simulink model "Copy_of_WorkshopB_1"  (R2014b)
settings: Solver=ode45  SolverMode=SingleTasking  StartTime=0.0  StopTime=5  RelTol=1e-3
values from neighbouring files (symbols this model uses):
  dm = dm*eps_dm    (= 1.3528e-05)    [param.m]
  Dpos = double(D)    [param.m]
  Fc = 0.0013    [param.m]
  Ipos = double(I)    [param.m]
  Jeq = eps_Jeq*Jeq    (= 2.20476e-05)    [param.m]
  Kemf = 1/(137*2*pi/60)    (= 0.0697028947848)    [param.m]
  Km = 69.7E-3    (= 0.0697)    [param.m]
  Max_Accel = Km*MaxCurrent/Jeq    (= 460.291369582)    [param.m]
  Max_Speed = MaxVoltage/Kemf    (= 275.454843867)    [param.m]
  n = 1    [param.m]
  Npos = double(N)    [param.m]
  Ppos = double(P)    [param.m]
  R = s*s + s*N    [PID_calc.m]    (also in param.m = 112)
  Ts = 5e-3    (= 0.005)    [param.m]
undefined symbols (not defined in the file or in its folder): sigbuilder_block
settings Model: Creator=sofianh  LastModifiedBy=es2lab2
settings OptimizationCC: BlockReduction=off  BooleanDataType=off  UseDivisionForNetSlopeComputation=off  SimCompilerOptimization=off
settings DebuggingCC: SaveWithParameterizedLinksMsg=none  UnderspecifiedInitializationDetection=Classic  MergeDetectMultiDrivingBlocksExec=none  SignalResolutionControl=TryResolveAllWithWarning  SolverPrmCheckMsg=none  FrameProcessingCompatibilityMsg=error  AllowSymbolicDim=off
settings HardwareCC: TargetUnknown=on
settings RTWCC: RTWCompilerOptimization=off
settings ConfigComp: CovMetricSettings=dw  CovHtmlReporting=on  CovSaveCumulativeToWorkspaceVar=on  CovSaveSingleToWorkspaceVar=on  CovModelRefEnable=Off  CovExternalEMLEnable=off  CovSFcnEnable=off

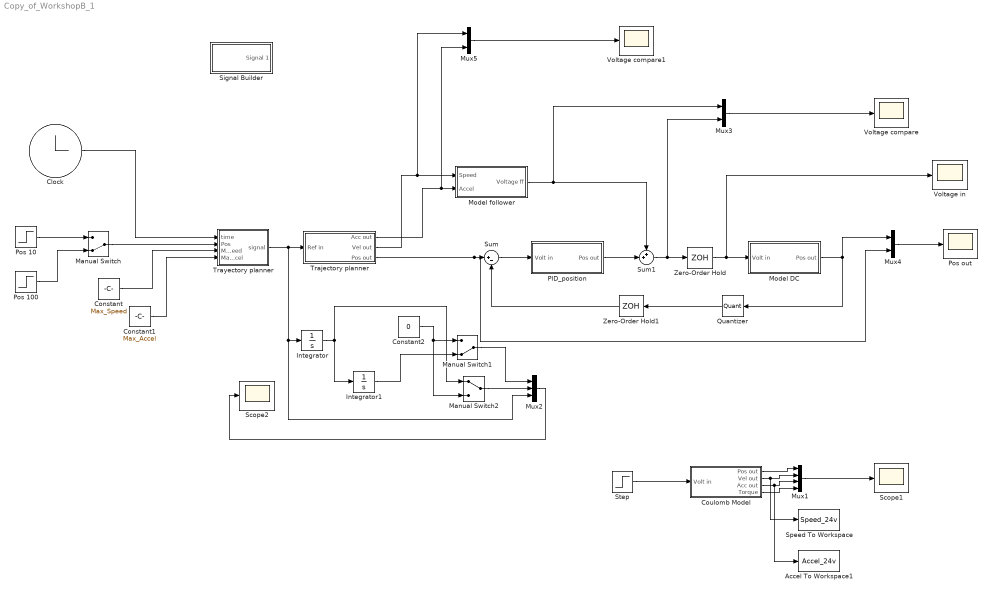
== system Copy_of_WorkshopB_1 ==
  Accel To Workspace1 : ToWorkspace  VariableName=Accel_24v  SaveFormat=Timeseries  SampleTime=-1
  Clock : Clock
  Constant : Constant  Value=Max_Speed
  Constant1 : Constant  Value=Max_Accel
  Constant2 : Constant  Value=0
  Coulomb Model : Subsystem
  Integrator : Integrator
  Integrator1 : Integrator
  Manual Switch : ManualSwitch  CurrentSetting=0
  Manual Switch1 : ManualSwitch  CurrentSetting=0
  Manual Switch2 : ManualSwitch
  "Model DC " : Subsystem
  Model follower : Subsystem
  Mux1 : Mux
  Mux2 : Mux  Inputs=3
  Mux3 : Mux  Inputs=2
  Mux4 : Mux  Inputs=2
  Mux5 : Mux  Inputs=2
  PID_position : Subsystem
  Pos 10 : Step  Time=0  After=10  SampleTime=0
  Pos 100 : Step  Time=0  After=100  SampleTime=0
  Pos out : Scope
      settings: TimeRange=4  SaveName=ScopeData3
  Quantizer : Quantizer  QuantizationInterval=Pulses  SampleTime=Ts
  Scope1 : Scope
  Scope2 : Scope
      settings: TimeRange=1  YMin=0  YMax=450
  Signal Builder : Subsystem  Tag=STV Subsys  LoadFcn=sigbuilder_block('load');  StartFcn=sigbuilder_block('start');  StopFcn=sigbuilder_block('stop');  ClipboardFcn=sigbuilder_block('clipboard');  mask(Sigbuilder block){}
      mask help: Simulink:masks:SigbuilderBlock_MD
      mask init:
      | if ~strcmp(get_param(bdroot(gcbh),'SimulationStatus'),'stopped') tuvar = sigbuilder_block('maskInit'); end
      settings: CopyFcn=sigbuilder_block('copy');  DeleteFcn=sigbuilder_block('delete');  ModelCloseFcn=sigbuilder_block('modelClose');  PreSaveFcn=sigbuilder_block('preSave');  PauseFcn=sigbuilder_block('pause');  ContinueFcn=sigbuilder_block('continue');  NameChangeFcn=sigbuilder_block('namechange');  OpenFcn=sigbuilder_block('open',[437.6 199.2 550.4 400 ]);  CloseFcn=sigbuilder_block('close');
      mask Display: plot(0, 0, 100, 100,[2, 2, 32, 32, 2], [68, 8, 8, 68, 68],[32, 2], [38, 38], [32, 19, 2],[53, 60, 44], [32, 17, 17, 2],[16, 16, 31, 31]);txt = getActiveGroup(gcbh);text(2, 100, txt,'verticalAlignment', 'top');
  Speed To Workspace : ToWorkspace  VariableName=Speed_24v  SaveFormat=Timeseries  SampleTime=-1
  Step : Step  Time=0  After=24  SampleTime=0
  Sum : Sum  Inputs=|+-
  Sum1 : Sum  Inputs=++|
  Trajectory planner : Subsystem
  Trayectory planner : MATLAB Function  TreatAsAtomicUnit=on  SystemSampleTime=Ts
  Voltage compare : Scope
      settings: SaveName=ScopeData2
  Voltage compare1 : Scope
      settings: SaveName=ScopeData6
  Voltage in : Scope
      settings: SaveName=ScopeData4
  Zero-Order Hold : ZeroOrderHold  SampleTime=Ts
  Zero-Order Hold1 : ZeroOrderHold  SampleTime=Ts
  wires:
  Mux1/1 -> Scope1/1
  Coulomb Model/1(Pos out) -> Mux1/1
  Step/1 -> Coulomb Model/1(Volt in)
  Coulomb Model/2(Vel out) -> Speed To Workspace/1, Mux1/2
  Coulomb Model/3(Acc out) -> Accel To Workspace1/1, Mux1/3
  Coulomb Model/4(Torque) -> Mux1/4
  Clock/1 -> Trayectory planner/1(time)
  Pos 10/1 -> Manual Switch/1
  Pos 100/1 -> Manual Switch/2
  Manual Switch/1 -> Trayectory planner/2(Pos)
  Integrator/1 -> Manual Switch2/1, Integrator1/1
  Integrator1/1 -> Manual Switch1/2
  Mux2/1 -> Scope2/1
  Constant/1 -> Trayectory planner/3(Max_Speed)
  Constant1/1 -> Trayectory planner/4(Max_Accel)
  Manual Switch1/1 -> Mux2/1
  Manual Switch2/1 -> Mux2/2
  Constant2/1 -> Manual Switch1/1, Manual Switch2/2
  Sum/1 -> PID_position/1(Volt in)
  "Model DC "/1(Pos out) -> Quantizer/1, Mux4/1
  PID_position/1(Pos out) -> Sum1/2
  Mux3/1 -> Voltage compare/1
  Model follower/1(Voltage ff) -> Sum1/1, Mux3/1
  Trayectory planner/1(signal) -> Mux2/3, Integrator/1, Trajectory planner/1(Ref in)
  Mux4/1 -> Pos out/1
  Trajectory planner/1("Acc out ") -> Mux5/2, Model follower/2(Accel)
  Mux5/1 -> Voltage compare1/1
  Trajectory planner/2(Vel out) -> Mux5/1, Model follower/1(Speed)
  Trajectory planner/3("Pos out ") -> Mux4/2, Sum/1
  Zero-Order Hold/1 -> Voltage in/1, "Model DC "/1("Volt in ")
  Sum1/1 -> Mux3/2, Zero-Order Hold/1
  Quantizer/1 -> Zero-Order Hold1/1
  Zero-Order Hold1/1 -> Sum/2

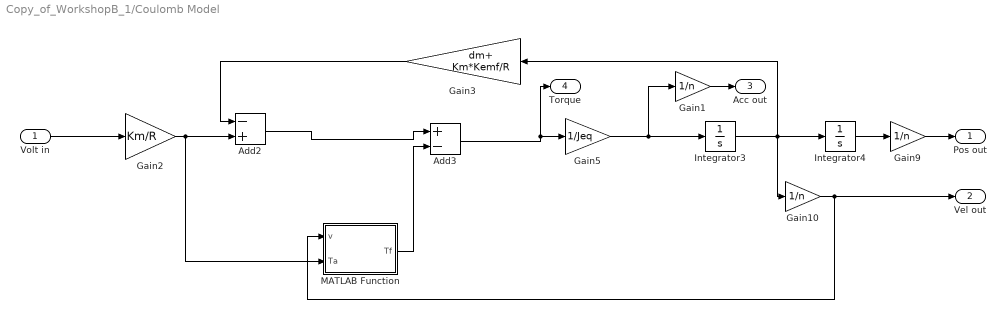
== system Copy_of_WorkshopB_1/Coulomb Model ==
  Volt in : Inport
  Add2 : Sum  Inputs=-+
  Add3 : Sum  Inputs=+-
  Gain1 : Gain  Gain=1/n
  Gain10 : Gain  Gain=1/n
  Gain2 : Gain  Gain=Km/R
  Gain3 : Gain  Gain=dm+ Km*Kemf/R
  Gain5 : Gain  Gain=1/Jeq
  Gain9 : Gain  Gain=1/n
  Integrator3 : Integrator
  Integrator4 : Integrator
  MATLAB Function : MATLAB Function  TreatAsAtomicUnit=on
  Pos out : Outport
  Vel out : Outport  Port=2
  Acc out : Outport  Port=3
  Torque : Outport  Port=4
  wires:
  Gain2/1 -> MATLAB Function/2(Ta), Add2/2
  Integrator3/1 -> Integrator4/1, Gain10/1, Gain3/1
  Gain3/1 -> Add2/1
  Gain5/1 -> Integrator3/1, Gain1/1
  Integrator4/1 -> Gain9/1
  Gain10/1 -> Vel out/1, MATLAB Function/1(v)
  Volt in/1 -> Gain2/1
  Add3/1 -> Torque/1, Gain5/1
  Add2/1 -> Add3/1
  MATLAB Function/1(Tf) -> Add3/2
  Gain9/1 -> Pos out/1
  Gain1/1 -> Acc out/1

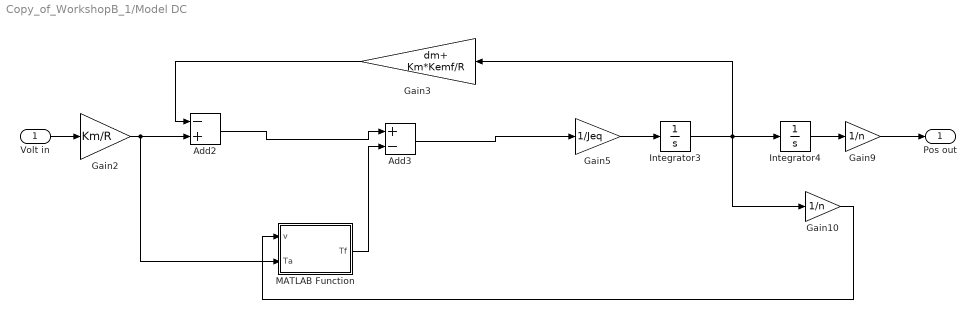
== system Copy_of_WorkshopB_1/Model DC  ==
  "Volt in " : Inport
  Add2 : Sum  Inputs=-+
  Add3 : Sum  Inputs=+-
  Gain10 : Gain  Gain=1/n
  Gain2 : Gain  Gain=Km/R
  Gain3 : Gain  Gain=dm+ Km*Kemf/R
  Gain5 : Gain  Gain=1/Jeq
  Gain9 : Gain  Gain=1/n
  Integrator3 : Integrator
  Integrator4 : Integrator
  MATLAB Function : MATLAB Function  TreatAsAtomicUnit=on
  Pos out : Outport
  wires:
  Gain2/1 -> MATLAB Function/2(Ta), Add2/2
  Integrator3/1 -> Integrator4/1, Gain10/1, Gain3/1
  Gain3/1 -> Add2/1
  Gain5/1 -> Integrator3/1
  Integrator4/1 -> Gain9/1
  Gain10/1 -> MATLAB Function/1(v)
  Add3/1 -> Gain5/1
  Add2/1 -> Add3/1
  MATLAB Function/1(Tf) -> Add3/2
  "Volt in "/1 -> Gain2/1
  Gain9/1 -> Pos out/1

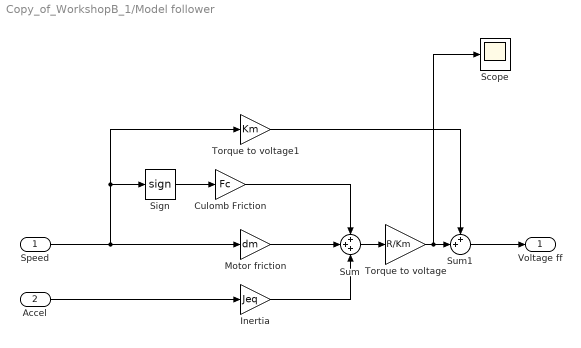
== system Copy_of_WorkshopB_1/Model follower ==
  Speed : Inport
  Accel : Inport  Port=2
  Culomb Friction : Gain  Gain=Fc
  "Inertia " : Gain  Gain=Jeq
  Motor friction : Gain  Gain=dm
  Scope : Scope
      settings: SaveName=ScopeData5
  Sign : Signum
  Sum : Sum  Inputs=+++
  Sum1 : Sum  Inputs=++|
  Torque to voltage : Gain  Gain=R/Km
  Torque to voltage1 : Gain  Gain=Km
  Voltage ff : Outport
  wires:
  Accel/1 -> "Inertia "/1
  Speed/1 -> Torque to voltage1/1, Sign/1, Motor friction/1
  "Inertia "/1 -> Sum/3
  Motor friction/1 -> Sum/2
  Sum/1 -> Torque to voltage/1
  Torque to voltage1/1 -> Sum1/1
  Torque to voltage/1 -> Scope/1, Sum1/2
  Sum1/1 -> Voltage ff/1
  Sign/1 -> Culomb Friction/1
  Culomb Friction/1 -> Sum/1

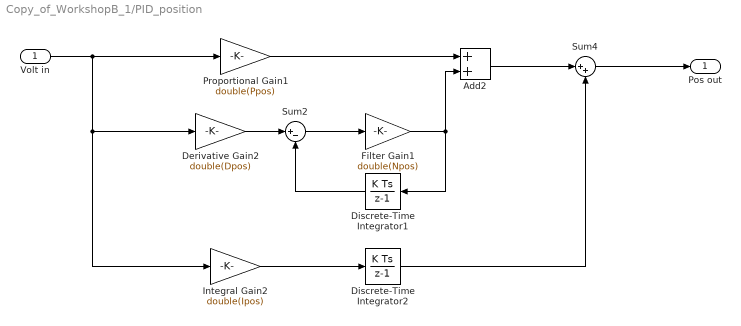
== system Copy_of_WorkshopB_1/PID_position ==
  Volt in : Inport
  Add2 : Sum
  Derivative Gain2 : Gain  Gain=double(Dpos)
  Discrete-Time Integrator1 : DiscreteIntegrator  InitialConditionSetting=State (most efficient)  SampleTime=Ts
  Discrete-Time Integrator2 : DiscreteIntegrator  InitialConditionSetting=State (most efficient)  SampleTime=Ts
  Filter Gain1 : Gain  Gain=double(Npos)
  Integral Gain2 : Gain  Gain=double(Ipos)
  Proportional Gain1 : Gain  Gain=double(Ppos)
  Sum2 : Sum  Inputs=|+-
  Sum4 : Sum  Inputs=|++
  Pos out : Outport
  wires:
  Discrete-Time Integrator2/1 -> Sum4/2
  Add2/1 -> Sum4/1
  Volt in/1 -> Integral Gain2/1, Derivative Gain2/1, Proportional Gain1/1
  Discrete-Time Integrator1/1 -> Sum2/2
  Sum2/1 -> Filter Gain1/1
  Derivative Gain2/1 -> Sum2/1
  Proportional Gain1/1 -> Add2/1
  Filter Gain1/1 -> Discrete-Time Integrator1/1, Add2/2
  Integral Gain2/1 -> Discrete-Time Integrator2/1
  Sum4/1 -> Pos out/1

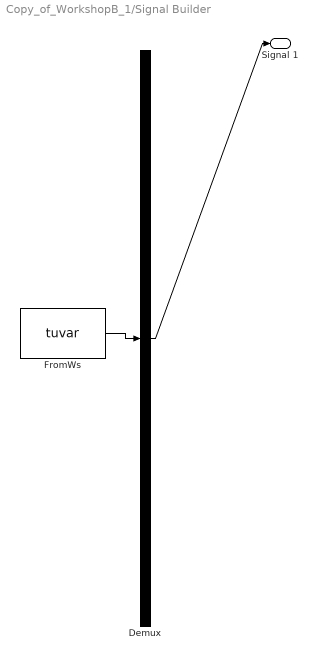
== system Copy_of_WorkshopB_1/Signal Builder ==
  Demux : Demux  Tag=STV Demux  Outputs=1
  FromWs : FromWorkspace  Tag=STV FromWs  VariableName=tuvar  SampleTime=0
      SigBuilderData=|
      | common.afterFinalStr = 'Extrapolate'
      | common.sampleTime = 0
      | dataSet.timeRange = [0 1]
      | dataSet.name = 'Group 1'
      | sbobj.Groups.Name = 'Group 1'
      | sbobj.Groups.Signals.Name = 'Signal 1'
      | sbobj.Groups.Signals.XData = [0 0.253892901991 0.253892901991 0.507785803983 0.507785803983 1]
      | sbobj.Groups.Signals.YData = [100 100 -100 -100 0 0]
      | sbobj.Groups.TimeRange = [0 1]
  Signal 1 : Outport  Tag=STV Outport
  wires:
  FromWs/1 -> Demux/1
  Demux/1 -> Signal 1/1

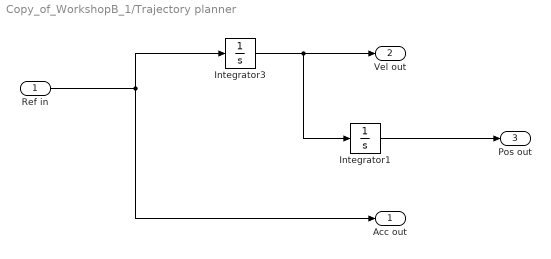
== system Copy_of_WorkshopB_1/Trajectory planner ==
  Ref in : Inport
  Integrator1 : Integrator
  Integrator3 : Integrator
  "Acc out " : Outport
  Vel out : Outport  Port=2
  "Pos out " : Outport  Port=3
  wires:
  Integrator3/1 -> Integrator1/1, Vel out/1
  Ref in/1 -> Integrator3/1, "Acc out "/1
  Integrator1/1 -> "Pos out "/1

== matlab function Copy_of_WorkshopB_1/Trayectory planner ==
  data: time input; signal output; Pos input; Max_Speed input; Max_Accel input
function signal = Planner(time,Pos,Max_Speed, Max_Accel)

trising = Max_Speed/Max_Accel;
Pos_rising = trising*0.5*Max_Speed;
%Max_Speed = Pos/(2*trising);
%Max_Accel = Max_Speed/trising;
t_est = (Pos - Max_Speed*trising)/Max_Speed;

    if time < trising
        signal = Max_Accel;
    elseif time >= trising && time < (trising + t_est)
        signal = 0; 
    elseif time >= (trising + t_est) && time < (2*trising + t_est)
        signal = - Max_Accel;
    else
        signal = 0;
    end

end

== matlab function Copy_of_WorkshopB_1/Coulomb Model/MATLAB Function ==
  data: v input; Tf output; Ta input
function Tf = fcn(v,Ta)
Tc = 1e-3;
dv = 1e-1;
if abs(v) < dv
    if abs(Ta) > Tc
        Tf = Tc*sign(Ta);
    else
        Tf = Ta;
    end
else
    Tf = Tc*sign(v);
end

== matlab function Copy_of_WorkshopB_1/Model DC /MATLAB Function ==
  data: v input; Tf output; Ta input
function Tf = fcn(v,Ta)
Tc = 1e-3;
dv = 1e-1;
if abs(v) < dv
    if abs(Ta) > Tc
        Tf = Tc*sign(Ta);
    else
        Tf = Ta;
    end
else
    Tf = Tc*sign(v);
end
